simulink subsystem "Attitude_Controller"  (R2025b)
settings: Solver=VariableStepAuto  StartTime=0.0  StopTime=10.0  RelTol=1e-3
libraries: matrix_library x1
settings Model: Creator=Kaan Kalkandelen  LastModifiedBy=Kaan Kalkandelen

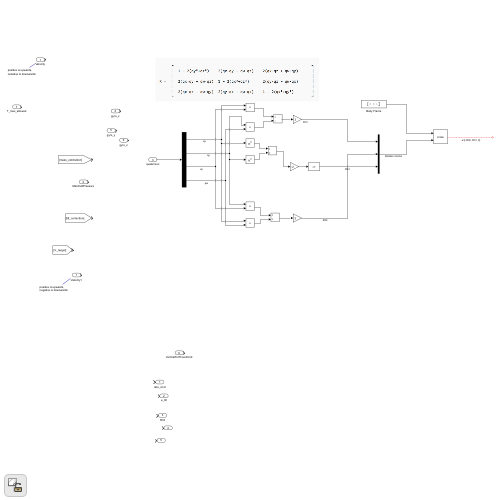
[thumbnail: Simulink's stored preview of the top-level diagram]
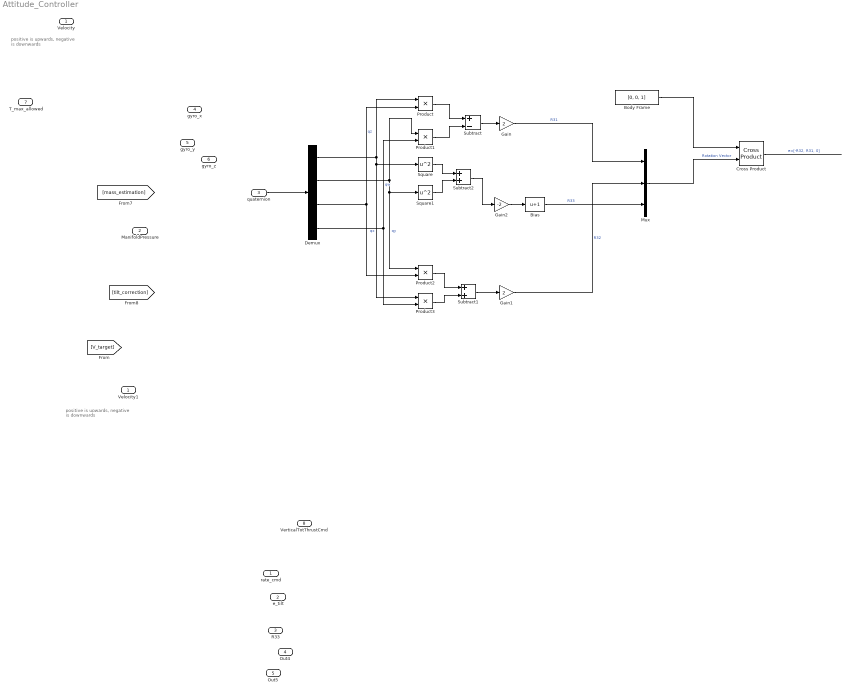
== system Attitude_Controller ==
  note: positive is upwards, negative is downwards
  note: positive is upwards, negative is downwards
  Velocity : Inport
  ManifoldPressure : Inport  Port=2
  quaternion : Inport  Port=3
  gyro_x : Inport  Port=4
  gyro_y : Inport  Port=5
  gyro_z : Inport  Port=6
  T_max_allowed : Inport  Port=7
  VerticalTotThrustCmd : Inport  Port=8
  Bias : Bias  Bias=1  SaturateOnIntegerOverflow=off
  Body Frame : Constant  Value=[0, 0, 1]
  Cross Product : matrix_library/Cross Product
  Demux : Demux
  Gain : Gain  Gain=2
  Gain1 : Gain  Gain=2
  Gain2 : Gain  Gain=-2
  Mux : Mux  Inputs=3
  Product{,1..3} (4 alike) : Product
  Square : Math  Operator=square
  Square1 : Math  Operator=square
  Subtract : Sum  Inputs=+-
  Subtract1 : Sum
  Subtract2 : Sum
  Velocity1 : InportShadow
  rate_cmd : Outport
  e_tilt : Outport  Port=2
  R33 : Outport  Port=3
  Out4 : Outport  Port=4
  Out5 : Outport  Port=5
  wires:
  quaternion/1 -> Demux/1
  Demux/1 -> Product/1, Square/1, Product3/1  "qx"
  Demux/2 -> Product1/1, Product2/1, Square1/1  "qy"
  Demux/3 -> Product/2, Product2/2  "qz"
  Demux/4 -> Product1/2, Product3/2  "qw"
  Product/1 -> Subtract/1
  Product1/1 -> Subtract/2
  Subtract/1 -> Gain/1
  Gain/1 -> Mux/1  "R31"
  Product2/1 -> Subtract1/1
  Product3/1 -> Subtract1/2
  Subtract1/1 -> Gain1/1
  Gain1/1 -> Mux/2  "R32"
  Body Frame/1 -> Cross Product/1
  Square/1 -> Subtract2/1
  Square1/1 -> Subtract2/2
  Subtract2/1 -> Gain2/1
  Gain2/1 -> Bias/1
  Bias/1 -> Mux/3  "R33"
  Mux/1 -> Cross Product/2  "Rotation Vector"
  Cross Product/1 -> ?  "e=[-R32, R31, 0]"
